simulink model "ZETAMPPTcomplete"  (R2017a)
settings: Solver=ode23tb  StartTime=0.0  StopTime=.2  FixedStep=1e-5  MaxStep=1e-4  RelTol=1e-3
libraries: powerlib x27, simulink x3, powerlib_extras x1, re_lib x1
settings Model: Creator=acer  LastModifiedBy=acer

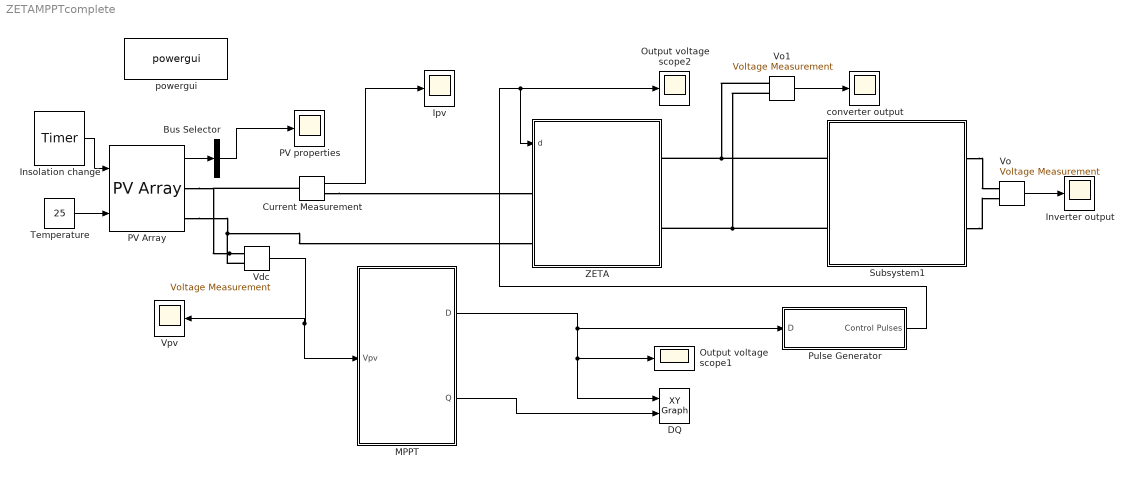
== system ZETAMPPTcomplete ==
  Bus Selector : BusSelector  OutputSignals=V_PV  OutputAsBus=on
  Current Measurement : powerlib/Measurements/Current Measurement  PhasorSimulation=off  OutputType=Complex  PSBequivalent=0
  DQ : simulink/Sinks/XY Graph  xmin=0  xmax=.1  ymin=0  ymax=.3  st=.0001
  Insolation change : powerlib_extras/Control  Blocks/Timer  t="[0  .1]"  e=[500 600]
  Inverter output : Scope
  Ipv : Scope
  MPPT : Subsystem
  Output voltage scope1 : Scope
  Output voltage scope2 : Scope
  PV Array : re_lib/Solar/PV Array  Npar=2  Nser=1  PlotType=one module @ 25 deg.C & specified irradiances  S_vec=[500 600]  Temp_C_vec="[ 45 25  ]"  ModuleName=User-defined  PlotWhenSelected=on  Pm=20.1544  Ncell=2  Voc=21.17  Isc=1.26  Vm=17.08  Im=1.18  beta_Voc_pc=-0.2941  alpha_Isc_pc=0.0681  beta_Voc=-0.062261  alpha_Isc=0.00085806  IL=1.2761  I0=3.4286e-12  nI=15.4858  Rsh=444.5152  Rs=1.4208  BAL=on  Tc=1e-6  Tfilter=2e-5
  PV properties : Scope
  Pulse Generator : Subsystem  mask{F=5e3}
      mask prompts: F "Carrier Frequency"
  Subsystem1 : Subsystem
  Temperature : Constant  Value=25  VectorParams1D=off  SampleTime=2e-5
  "Vdc " : powerlib/Measurements/Voltage Measurement  Tag=PoWeRsYsTeMmEaSuReMeNt  PhasorSimulation=off  OutputType=Magnitude  PSBequivalent=0
  Vo : powerlib/Measurements/Voltage Measurement  PhasorSimulation=off  OutputType=Complex  PSBequivalent=0
  Vo1 : powerlib/Measurements/Voltage Measurement  PhasorSimulation=off  OutputType=Complex  PSBequivalent=0
  Vpv : Scope
  ZETA : Subsystem
  converter output : Scope
  powergui : powerlib/powergui  Priority=1  SimulationMode=Discrete  SampleTime=50e-6  frequency=50  Iterations=50  frequencyindice=0  Pbase=100e6  ErrMax=1e-4  UnitsV=kV  UnitsW=MW  buscounter=0  FunctionMessages=off  echomessages=off  EnableUseOfTLC=off  CurrentSourceSwitches=off  DisableSnubberDevices=off  DisableRonSwitches=off  DisableVfSwitches=off  DisplayEquations=off  SolverType=Tustin/Backward Euler (TBE)  Interpol=off  ExternalGateDelay=off  methode=off  Ts=100  x0status=blocks  SPID=on  SwTol=0  HookPort=off  RestoreLinks=warning  ResistiveCurrentMeasurement=off  Frange=[0:2:500]  Ylog=off  Xlog=on  ShowGrid=off  save=off  variable=ZData  structure=inverterOutputMPPT  ZoomFFT=off  StartTime=0  cycles=10  DisplayStyle=1  fundamental=50  FreqAxis=off  MaxFrequency=1000  frequencyindicesteady=1  RmsSteady=1  display=off
  wires:
  Temperature/1 -> PV Array/2
  PV Array/1 -> Bus Selector/1
  Bus Selector/1 -> PV properties/1
  Insolation change/1 -> PV Array/1
  Current Measurement/1 -> Ipv/1
  Pulse Generator/1(Control Pulses) -> ZETA/1(d), Output voltage scope2/1
  "Vdc "/1 -> MPPT/1(Vpv), Vpv/1
  MPPT/2(Q) -> DQ/2
  MPPT/1(D) -> DQ/1, Output voltage scope1/1, Pulse Generator/1(D)
  Vo/1 -> Inverter output/1
  Vo1/1 -> converter output/1
  connections:
  "Vdc "/LConn1 -- PV Array/RConn1 -- Current Measurement/LConn1
  "Vdc "/LConn2 -- PV Array/RConn2 -- ZETA/LConn2
  Current Measurement/RConn1 -- ZETA/LConn1
  Subsystem1/LConn1 -- Vo1/LConn1 -- ZETA/RConn1
  Subsystem1/LConn2 -- Vo1/LConn2 -- ZETA/RConn2
  Subsystem1/RConn1 -- Vo/LConn1
  Subsystem1/RConn2 -- Vo/LConn2

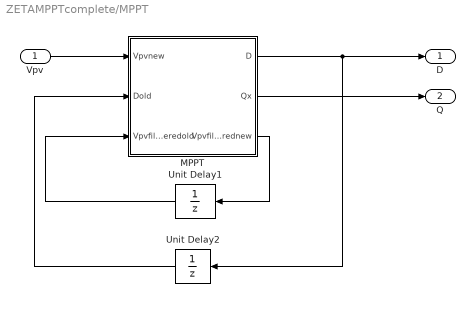
== system ZETAMPPTcomplete/MPPT ==
  Vpv : Inport
  MPPT : MATLAB Function  TreatAsAtomicUnit=on
  Unit Delay1 : UnitDelay  SampleTime=.0001
  Unit Delay2 : UnitDelay  SampleTime=.0001
  D : Outport
  Q : Outport  Port=2
  wires:
  MPPT/1(D) -> D/1, Unit Delay2/1
  Vpv/1 -> MPPT/1(Vpvnew)
  MPPT/2(Qx) -> Q/1
  Unit Delay2/1 -> MPPT/2(Dold)
  Unit Delay1/1 -> MPPT/3(Vpvfilteredold)
  MPPT/3(Vpvfilterednew) -> Unit Delay1/1

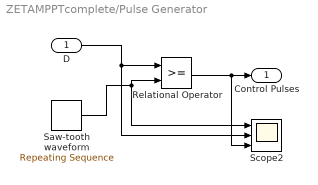
== system ZETAMPPTcomplete/Pulse Generator ==
  D : Inport
  Relational Operator : RelationalOperator  OutDataTypeStr=boolean  RndMeth=Nearest
  Saw-tooth waveform : simulink/Sources/Repeating Sequence  rep_seq_t=[0 0.5 1]/F  rep_seq_y=[0 1 0]
  Scope2 : Scope  NumInputPorts=3
  Control Pulses : Outport
  wires:
  Saw-tooth waveform/1 -> Relational Operator/2, Scope2/1
  Relational Operator/1 -> Scope2/3, Control Pulses/1
  D/1 -> Relational Operator/1, Scope2/2

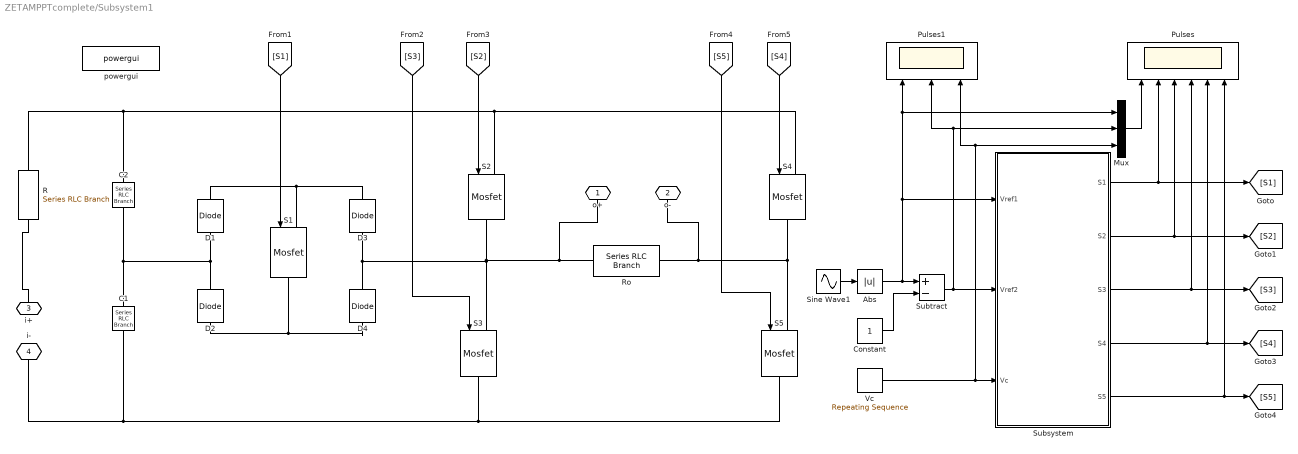
== system ZETAMPPTcomplete/Subsystem1 ==
  Abs : Abs
  C1 : powerlib/Elements/Series RLC Branch  LConnTagsString=__new0  RConnTagsString=__new0  BranchType=C  Resistance=100  Inductance=1e-3  SetiL0=off  InitialCurrent=0  Capacitance=2  Setx0=on  InitialVoltage=10  Measurements=None
  C2 : powerlib/Elements/Series RLC Branch  LConnTagsString=__new0  RConnTagsString=__new0  BranchType=C  Resistance=100  Inductance=1e-3  SetiL0=off  InitialCurrent=0  Capacitance=2  Setx0=on  InitialVoltage=10  Measurements=None
  Constant : Constant
  D{1..4} (4 alike) : powerlib/Power Electronics/Diode  Ron=0.001  Lon=0  Vf=.05  IC=0  UseSnubber=off  Rs=500  Cs=250e-9  Measurements=off
  Mux : Mux  Inputs=3
  Pulses : Scope  NumInputPorts=6
  Pulses1 : Scope  NumInputPorts=3
  R : powerlib/Elements/Series RLC Branch  LConnTagsString=__new0  RConnTagsString=__new0  BranchType=R  Resistance=1e-8  Inductance=1e-3  SetiL0=off  InitialCurrent=0  Capacitance=1e-6  Setx0=off  InitialVoltage=0  Measurements=None
  Ro : powerlib/Elements/Series RLC Branch  LConnTagsString=__new0  RConnTagsString=__new0  BranchType=R  Resistance=5  Inductance=1e-3  SetiL0=off  InitialCurrent=0  Capacitance=1e-6  Setx0=off  InitialVoltage=0  Measurements=None
  S{1..5} (5 alike) : powerlib/Power Electronics/Mosfet  Ron=0.1  Lon=0  Rd=0.01  Vfd=0  IC=0  Rs=1e5  Cs=inf  Measurements=off
  Sine Wave1 : Sin  Amplitude=2.5  Frequency=2*pi*50  SampleTime=0  VectorParams1D=off
  Subsystem : Subsystem
  Subtract : Sum  Inputs=+-
  Vc : simulink/Sources/Repeating Sequence  rep_seq_t="[0  1e-5 2e-5]"  rep_seq_y=[0 1 0]
  powergui : powerlib/powergui  Priority=1  SimulationMode=Continuous  SampleTime=1e-6  frequency=60  Iterations=50  frequencyindice=0  Pbase=100e6  ErrMax=1e-4  UnitsV=kV  UnitsW=MW  buscounter=0  FunctionMessages=off  echomessages=off  EnableUseOfTLC=off  CurrentSourceSwitches=off  DisableSnubberDevices=off  DisableRonSwitches=off  DisableVfSwitches=off  DisplayEquations=off  SolverType=Tustin/Backward Euler (TBE)  Interpol=off  ExternalGateDelay=off  methode=off  Ts=100  x0status=blocks  SPID=on  SwTol=0  HookPort=off  RestoreLinks=warning  ResistiveCurrentMeasurement=off  Frange=[0:2:500]  Ylog=off  Xlog=on  ShowGrid=off  save=off  variable=ZData  structure=outputVoltage  ZoomFFT=off  StartTime=0  cycles=10  DisplayStyle=3  fundamental=50  FreqAxis=off  MaxFrequency=1000  frequencyindicesteady=1  RmsSteady=1  display=off
  o+ : PMIOPort  Port=1  Side=Right
  o- : PMIOPort  Port=2  Side=Right
  i+ : PMIOPort  Port=3  Side=Left
  i- : PMIOPort  Port=4  Side=Left
  wires:
  Abs/1 -> Mux/1, Pulses1/1, Subsystem/1(Vref1), Subtract/1
  [S1] -> S1/1
  Subsystem/5(S5) -> [S5], Pulses/6
  Subsystem/4(S4) -> [S4], Pulses/5
  [S3] -> S3/1
  Sine Wave1/1 -> Abs/1
  Subsystem/2(S2) -> [S2], Pulses/3
  [S4] -> S4/1
  Subsystem/3(S3) -> [S3], Pulses/4
  [S2] -> S2/1
  Subsystem/1(S1) -> [S1], Pulses/2
  Subtract/1 -> Subsystem/2(Vref2), Pulses1/2, Mux/2
  Constant/1 -> Subtract/2
  Mux/1 -> Pulses/1
  Vc/1 -> Subsystem/3(Vc), Pulses1/3, Mux/3
  [S5] -> S5/1
  connections:
  S1/LConn1 -- D3/RConn1 -- D1/RConn1
  S4/LConn1 -- S2/LConn1 -- R/RConn1 -- C2/LConn1
  C1/RConn1 -- S3/RConn1 -- S5/RConn1 -- i-/RConn1
  Ro/LConn1 -- S2/RConn1 -- D3/LConn1 -- D4/RConn1 -- S3/LConn1 -- o+/RConn1
  Ro/RConn1 -- S4/RConn1 -- S5/LConn1 -- o-/RConn1
  S1/RConn1 -- D2/LConn1 -- D4/LConn1
  R/LConn1 -- i+/RConn1
  C2/RConn1 -- D2/RConn1 -- D1/LConn1 -- C1/LConn1

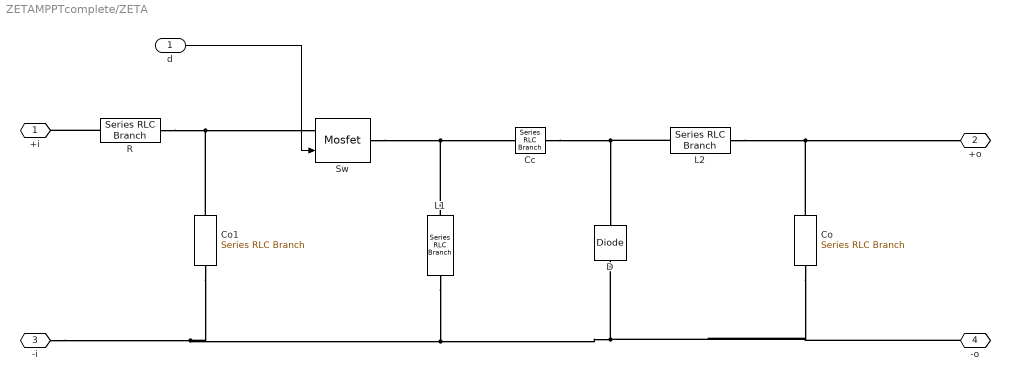
== system ZETAMPPTcomplete/ZETA ==
  d : Inport
  Cc : powerlib/Elements/Series RLC Branch  LConnTagsString=__new0  RConnTagsString=__new0  BranchType=C  Resistance=100  Inductance=1e-3  SetiL0=off  InitialCurrent=0  Capacitance=60e-6  Setx0=off  InitialVoltage=17  Measurements=None
  Co : powerlib/Elements/Series RLC Branch  LConnTagsString=__new0  RConnTagsString=__new0  BranchType=C  Resistance=1  Inductance=1e-3  SetiL0=off  InitialCurrent=0  Capacitance=1e-3  Setx0=on  InitialVoltage=20  Measurements=None
  Co1 : powerlib/Elements/Series RLC Branch  LConnTagsString=__new0  RConnTagsString=__new0  BranchType=C  Resistance=1  Inductance=1e-3  SetiL0=off  InitialCurrent=0  Capacitance=1e-3  Setx0=on  InitialVoltage=15  Measurements=None
  D : powerlib/Power Electronics/Diode  Ron=0.001  Lon=0  Vf=.05  IC=0  UseSnubber=off  Rs=500  Cs=250e-9  Measurements=off
  L1 : powerlib/Elements/Series RLC Branch  LConnTagsString=__new0  RConnTagsString=__new0  BranchType=L  Resistance=1  Inductance=300e-6  SetiL0=off  InitialCurrent=1  Capacitance=1e-6  Setx0=off  InitialVoltage=0  Measurements=None
  L2 : powerlib/Elements/Series RLC Branch  LConnTagsString=__new0  RConnTagsString=__new0  BranchType=L  Resistance=1  Inductance=300e-6  SetiL0=off  InitialCurrent=1  Capacitance=1e-6  Setx0=off  InitialVoltage=0  Measurements=None
  R : powerlib/Elements/Series RLC Branch  LConnTagsString=__new0  RConnTagsString=__new0  BranchType=R  Resistance=1e-12  Inductance=1e-3  SetiL0=off  InitialCurrent=0  Capacitance=1e-6  Setx0=off  InitialVoltage=0  Measurements=None
  Sw : powerlib/Power Electronics/Mosfet  Ron=0.1  Lon=0  Rd=0.01  Vfd=0  IC=0  Rs=1e5  Cs=inf  Measurements=off
  +i : PMIOPort  Port=1  Side=Left
  +o : PMIOPort  Port=2  Side=Right
  -i : PMIOPort  Port=3  Side=Left
  -o : PMIOPort  Port=4  Side=Right
  wires:
  d/1 -> Sw/1
  connections:
  -i/RConn1 -- L1/RConn1 -- D/LConn1 -- Co/RConn1 -- -o/RConn1 -- Co1/RConn1
  Co1/LConn1 -- Sw/LConn1 -- R/RConn1
  Sw/RConn1 -- L1/LConn1 -- Cc/LConn1
  Co/LConn1 -- +o/RConn1 -- L2/RConn1
  Cc/RConn1 -- L2/LConn1 -- D/RConn1
  R/LConn1 -- +i/RConn1

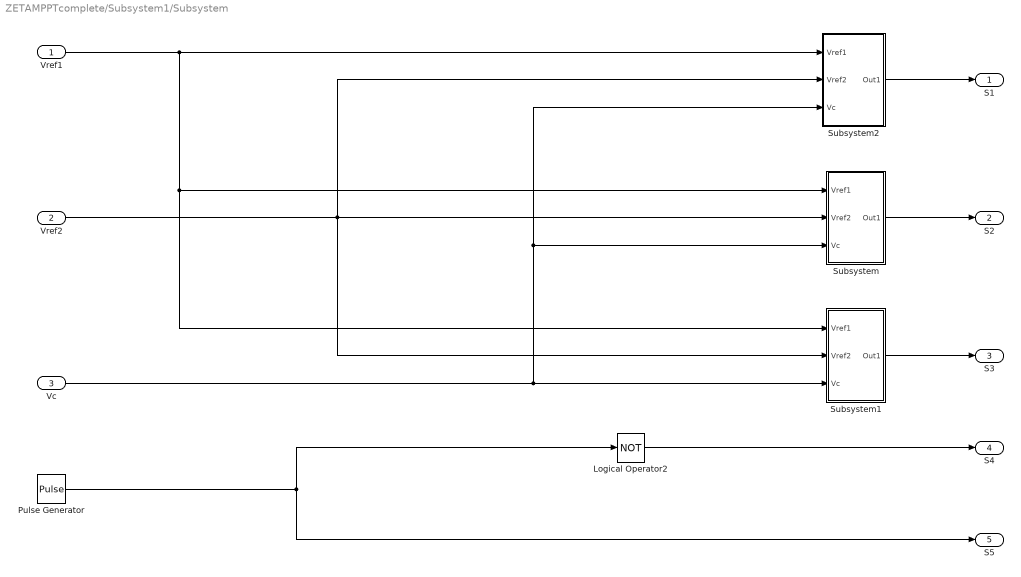
== system ZETAMPPTcomplete/Subsystem1/Subsystem ==
  Vref1 : Inport
  Vref2 : Inport  Port=2
  Vc : Inport  Port=3
  Logical Operator2 : Logic  Operator=NOT  AllPortsSameDT=off  OutDataTypeStr=boolean
  Pulse Generator : DiscretePulseGenerator  PulseType=Time based  Period=.02  PulseWidth=50
  Subsystem : Subsystem
  Subsystem1 : Subsystem
  Subsystem2 : Subsystem
  S1 : Outport
  S2 : Outport  Port=2
  S3 : Outport  Port=3
  S4 : Outport  Port=4
  S5 : Outport  Port=5
  wires:
  Subsystem1/1(Out1) -> S3/1
  Pulse Generator/1 -> Logical Operator2/1, S5/1
  Logical Operator2/1 -> S4/1
  Subsystem/1(Out1) -> S2/1
  Subsystem2/1(Out1) -> S1/1
  Vref1/1 -> Subsystem1/1(Vref1), Subsystem/1(Vref1), Subsystem2/1(Vref1)
  Vref2/1 -> Subsystem2/2(Vref2), Subsystem1/2(Vref2), Subsystem/2(Vref2)
  Vc/1 -> Subsystem2/3(Vc), Subsystem/3(Vc), Subsystem1/3(Vc)

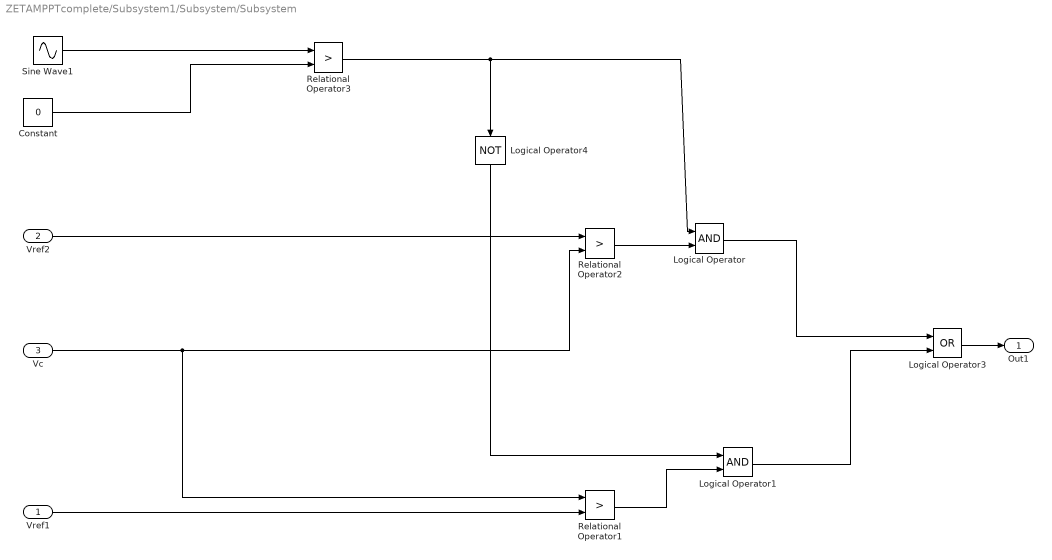
== system ZETAMPPTcomplete/Subsystem1/Subsystem/Subsystem ==
  Vref1 : Inport
  Vref2 : Inport  Port=2
  Vc : Inport  Port=3
  Constant : Constant  Value=0
  Logical Operator : Logic  AllPortsSameDT=off  OutDataTypeStr=boolean
  Logical Operator1 : Logic  AllPortsSameDT=off  OutDataTypeStr=boolean
  Logical Operator3 : Logic  Operator=OR  AllPortsSameDT=off  OutDataTypeStr=boolean
  Logical Operator4 : Logic  Operator=NOT  AllPortsSameDT=off  OutDataTypeStr=boolean
  Relational Operator1 : RelationalOperator  Operator=>  OutDataTypeStr=boolean  RndMeth=Nearest
  Relational Operator2 : RelationalOperator  Operator=>  OutDataTypeStr=boolean  RndMeth=Nearest
  Relational Operator3 : RelationalOperator  Operator=>  OutDataTypeStr=boolean  RndMeth=Nearest
  Sine Wave1 : Sin  Amplitude=100  Frequency=2*pi*50  SampleTime=0  VectorParams1D=off
  Out1 : Outport
  wires:
  Vref1/1 -> Relational Operator1/2
  Vref2/1 -> Relational Operator2/1
  Vc/1 -> Relational Operator1/1, Relational Operator2/2
  Relational Operator2/1 -> Logical Operator/2
  Logical Operator4/1 -> Logical Operator1/1
  Relational Operator1/1 -> Logical Operator1/2
  Logical Operator/1 -> Logical Operator3/1
  Logical Operator1/1 -> Logical Operator3/2
  Logical Operator3/1 -> Out1/1
  Sine Wave1/1 -> Relational Operator3/1
  Constant/1 -> Relational Operator3/2
  Relational Operator3/1 -> Logical Operator/1, Logical Operator4/1

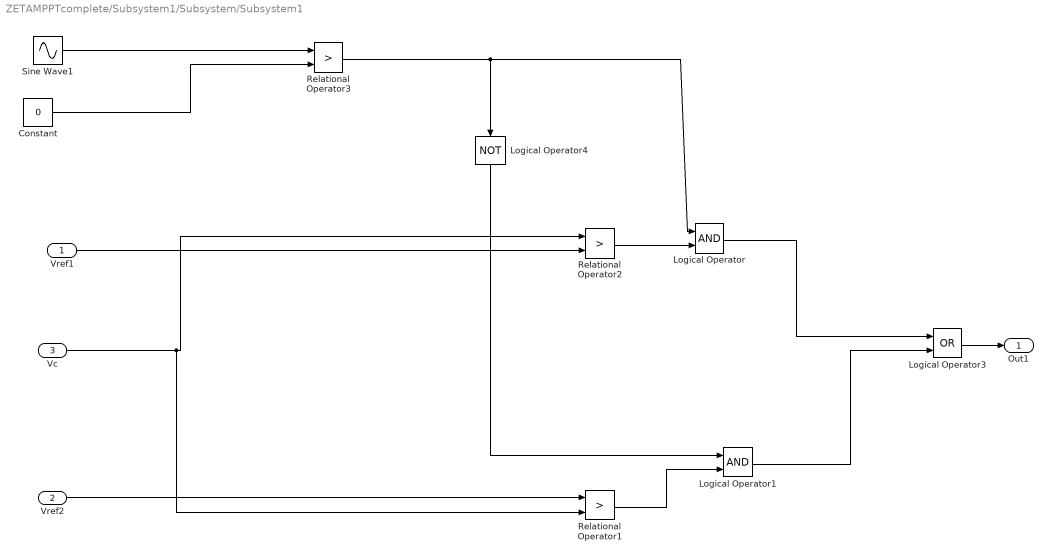
== system ZETAMPPTcomplete/Subsystem1/Subsystem/Subsystem1 ==
  Vref1 : Inport
  Vref2 : Inport  Port=2
  Vc : Inport  Port=3
  Constant : Constant  Value=0
  Logical Operator : Logic  AllPortsSameDT=off  OutDataTypeStr=boolean
  Logical Operator1 : Logic  AllPortsSameDT=off  OutDataTypeStr=boolean
  Logical Operator3 : Logic  Operator=OR  AllPortsSameDT=off  OutDataTypeStr=boolean
  Logical Operator4 : Logic  Operator=NOT  AllPortsSameDT=off  OutDataTypeStr=boolean
  Relational Operator1 : RelationalOperator  Operator=>  OutDataTypeStr=boolean  RndMeth=Nearest
  Relational Operator2 : RelationalOperator  Operator=>  OutDataTypeStr=boolean  RndMeth=Nearest
  Relational Operator3 : RelationalOperator  Operator=>  OutDataTypeStr=boolean  RndMeth=Nearest
  Sine Wave1 : Sin  Amplitude=100  Frequency=2*pi*50  SampleTime=0  VectorParams1D=off
  Out1 : Outport
  wires:
  Vref1/1 -> Relational Operator2/2
  Vc/1 -> Relational Operator1/2, Relational Operator2/1
  Relational Operator2/1 -> Logical Operator/2
  Logical Operator4/1 -> Logical Operator1/1
  Relational Operator1/1 -> Logical Operator1/2
  Logical Operator/1 -> Logical Operator3/1
  Logical Operator1/1 -> Logical Operator3/2
  Logical Operator3/1 -> Out1/1
  Sine Wave1/1 -> Relational Operator3/1
  Constant/1 -> Relational Operator3/2
  Relational Operator3/1 -> Logical Operator/1, Logical Operator4/1
  Vref2/1 -> Relational Operator1/1

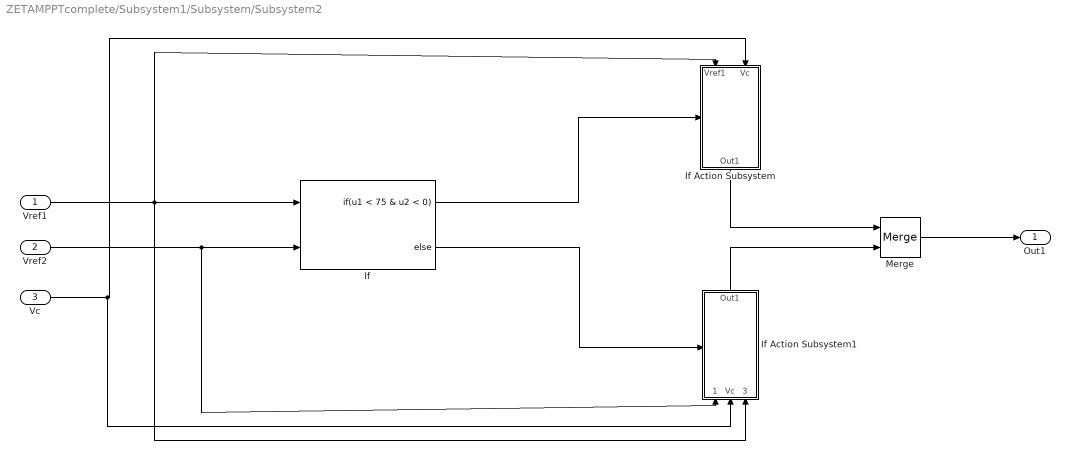
== system ZETAMPPTcomplete/Subsystem1/Subsystem/Subsystem2 ==
  Vref1 : Inport
  Vref2 : Inport  Port=2
  Vc : Inport  Port=3
  If : If  NumInputs=2  IfExpression=u1 < 75 & u2 < 0
  If Action Subsystem : Subsystem  TreatAsAtomicUnit=on
  If Action Subsystem1 : Subsystem  TreatAsAtomicUnit=on
  Merge : Merge
  Out1 : Outport
  wires:
  Vref1/1 -> If Action Subsystem1/3(Vref1), If/1, If Action Subsystem/1(Vref1)
  Merge/1 -> Out1/1
  Vref2/1 -> If Action Subsystem1/1(Vref2), If/2
  If/2 -> If Action Subsystem1/Action
  If/1 -> If Action Subsystem/Action
  If Action Subsystem/1(Out1) -> Merge/1
  If Action Subsystem1/1(Out1) -> Merge/2
  Vc/1 -> If Action Subsystem1/2(Vc), If Action Subsystem/2(Vc)

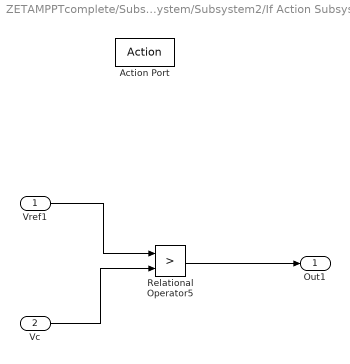
== system ZETAMPPTcomplete/Subsystem1/Subsystem/Subsystem2/If Action Subsystem ==
  Vref1 : Inport
  Vc : Inport  Port=2
  Action Port : ActionPort  ActionType=then
  Relational Operator5 : RelationalOperator  Operator=>  OutDataTypeStr=boolean  RndMeth=Nearest
  Out1 : Outport
  wires:
  Vref1/1 -> Relational Operator5/1
  Vc/1 -> Relational Operator5/2
  Relational Operator5/1 -> Out1/1

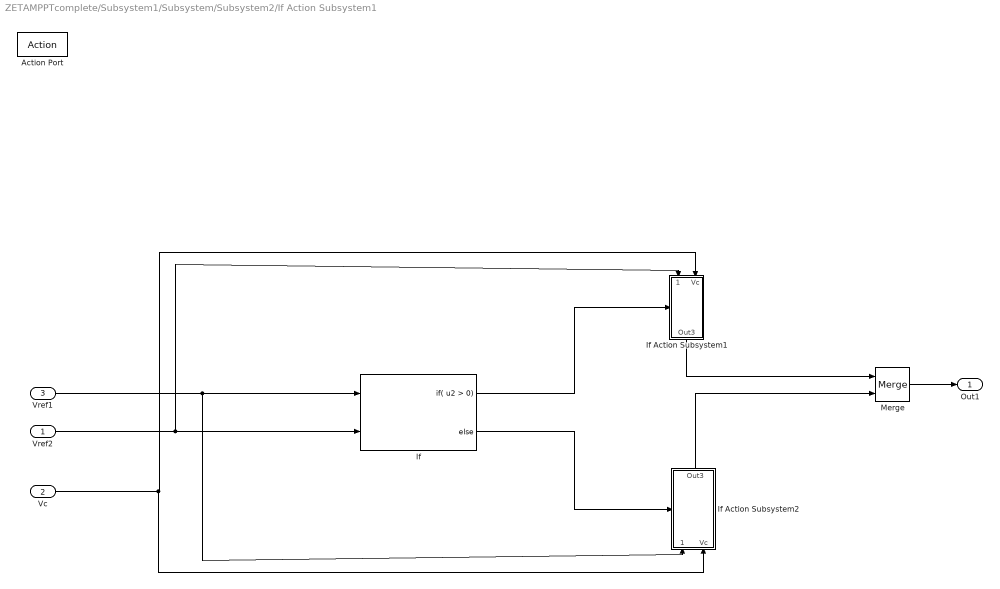
== system ZETAMPPTcomplete/Subsystem1/Subsystem/Subsystem2/If Action Subsystem1 ==
  Vref2 : Inport
  Vc : Inport  Port=2
  Vref1 : Inport  Port=3
  Action Port : ActionPort  ActionType=else
  If : If  NumInputs=2  IfExpression=u2 > 0
  If Action Subsystem1 : Subsystem  TreatAsAtomicUnit=on
  If Action Subsystem2 : Subsystem  TreatAsAtomicUnit=on
  Merge : Merge
  Out1 : Outport
  wires:
  Vref1/1 -> If Action Subsystem2/1(Vref1), If/1
  Vref2/1 -> If Action Subsystem1/1(Vref2), If/2
  If/1 -> If Action Subsystem1/Action
  If/2 -> If Action Subsystem2/Action
  If Action Subsystem1/1(Out3) -> Merge/1
  If Action Subsystem2/1(Out3) -> Merge/2
  Merge/1 -> Out1/1
  Vc/1 -> If Action Subsystem2/2(Vc), If Action Subsystem1/2(Vc)

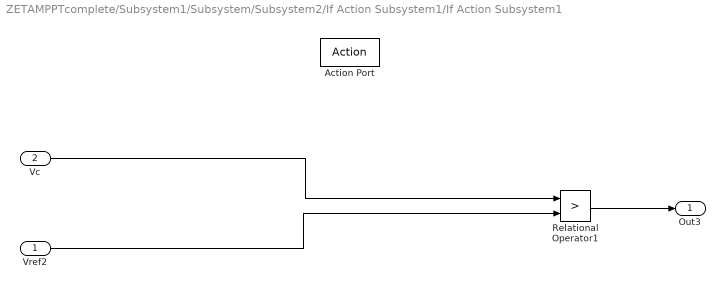
== system ZETAMPPTcomplete/Subsystem1/Subsystem/Subsystem2/If Action Subsystem1/If Action Subsystem1 ==
  Vref2 : Inport
  Vc : Inport  Port=2
  Action Port : ActionPort  ActionType=then
  Relational Operator1 : RelationalOperator  Operator=>  OutDataTypeStr=boolean  RndMeth=Nearest
  Out3 : Outport
  wires:
  Relational Operator1/1 -> Out3/1
  Vc/1 -> Relational Operator1/1
  Vref2/1 -> Relational Operator1/2

== system ZETAMPPTcomplete/Subsystem1/Subsystem/Subsystem2/If Action Subsystem1/If Action Subsystem2 ==
  Vref1 : Inport
  Vc : Inport  Port=2
  Action Port : ActionPort  ActionType=else
  Relational Operator1 : RelationalOperator  Operator=>  OutDataTypeStr=boolean  RndMeth=Nearest
  Out3 : Outport
  wires:
  Relational Operator1/1 -> Out3/1
  Vref1/1 -> Relational Operator1/1
  Vc/1 -> Relational Operator1/2

== matlab function ZETAMPPTcomplete/MPPT/MPPT ==
  data: Vpvnew input; Dold input; D output; Qx output; Vpvfilteredold input; Vpvfilterednew output
function [D,Qx,Vpvfilterednew]  = MPPT(Vpvnew,Dold,Vpvfilteredold)
%function [D,Qx,Vpvfilterednew,Ipvfilterednew,Ppv,delVpvnew,delPpv]  = MPPT( Ipvnew, Vpvnew,Dold,Vpvfilteredold,Ipvfilteredold,Ppvold,delVpvold,delPpvold)

Tdel = 1/(25e3);
t = 15.9e-3;
a = (Tdel/(Tdel+t));
Vpvfilterednew = ((Vpvfilteredold*(a-1))+(a*(Vpvnew)));

% Ipvfilterednew = ((Ipvfilteredold*(a-1))+(a*(Ipvnew)));
% Kp=100;
% Ki=.9;
% Ppv = Vpvfilterednew * Ipvfilterednew;
% delPpv = Ppvold - Ppv;
% delVpvnew = delVpvold + Kp * (delPpv - delPpvold) + (Ki * Tdel * delPpv );
delVpvnew = Vpvfilterednew -Vpvfilteredold;
M1=.0001;
M2=1  ;
%Dmax = .409416581
% Qth = (.409416581*(1-.409416581)*.0003))+(17*.0001)
Qth = 8.507e-3;

Ddel = 5e-2;
Qx=((1-Dold)* delVpvnew)+(Vpvnew*Ddel);
Q=abs(Qx);
if (Q>=Qth)
    dD = M1*Q;
else
    dD = M2*Q;
end
disp(Q);
if (Qx>0)
    D = Dold+dD;
elseif (Qx<0)
    D = Dold-dD;
else
    D = Dold;
end
